simulink model "motor_model_sl"  (R2015a)
settings: Solver=ode4  StartTime=0.0  StopTime=Tstop  FixedStep=T  RelTol=1e-3
settings Model: Creator=nguye  LastModifiedBy=nguye

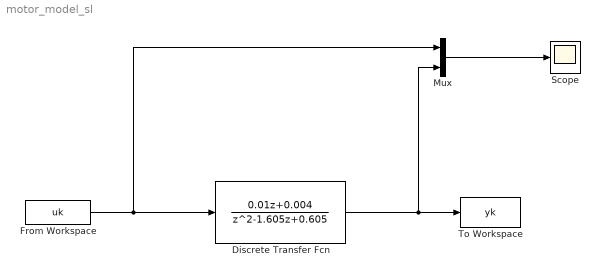
== system motor_model_sl ==
  Discrete Transfer Fcn : DiscreteTransferFcn  Numerator=[0.01 0.004]  Denominator=[1 -1.605 0.605]  SampleTime=0.01
  From Workspace : FromWorkspace  VariableName=uk  SampleTime=0.01
  Mux : Mux  Inputs=2
  Scope : Scope
  To Workspace : ToWorkspace  VariableName=yk  SampleTime=0.01
  wires:
  From Workspace/1 -> Mux/1, Discrete Transfer Fcn/1
  Discrete Transfer Fcn/1 -> Mux/2, To Workspace/1
  Mux/1 -> Scope/1
